simulink model "SG__REF_O_104"  (R2022b)
settings: Solver=FixedStepAuto  StartTime=0.0  StopTime=Inf  RelTol=1e-3  EnableMultiTasking=on
model workspace (MAT data in the model file):
  N_trig = Simulink.Parameter
  N_trig.Value = 4
  N_trig.Description = 'number of samples for triggered pulse for recording'
  N_trig.DataType = 'auto'
  N_trig.Complexity = 'real'
  N_trig.Dimensions = [1 1]
  a_1 = Simulink.Parameter
  a_1.Value = [1 1 1]
  a_1.DataType = 'auto'
  a_1.Complexity = 'real'
  a_1.Dimensions = [1 3]
  b_1 = Simulink.Parameter
  b_1.Value = [0.5 0.5 0.5]
  b_1.DataType = 'auto'
  b_1.Complexity = 'real'
  b_1.Dimensions = [1 3]
  enable_source = Simulink.Parameter
  enable_source.Value = 0
  enable_source.DataType = 'boolean'
  enable_source.Complexity = 'real'
  enable_source.Dimensions = [1 1]
  freq_fin = Simulink.Parameter
  freq_fin.Value = 1200
  freq_fin.DataType = 'auto'
  freq_fin.Complexity = 'real'
  freq_fin.Dimensions = [1 1]
  freq_ini = Simulink.Parameter
  freq_ini.Value = 150
  freq_ini.DataType = 'auto'
  freq_ini.Complexity = 'real'
  freq_ini.Dimensions = [1 1]
  k_1 = Simulink.Parameter
  k_1.Value = [0 0 0]
  k_1.DataType = 'auto'
  k_1.Complexity = 'real'
  k_1.Dimensions = [1 3]
  rec = Simulink.Parameter
  rec.Value = 0
  rec.DataType = 'boolean'
  rec.Complexity = 'real'
  rec.Dimensions = [1 1]
  src_select = Simulink.Parameter
  src_select.Value = 0
  src_select.DataType = 'auto'
  src_select.Complexity = 'real'
  src_select.Dimensions = [1 1]
  sweep_gain = Simulink.Parameter
  sweep_gain.Value = 0.02
  sweep_gain.DataType = 'auto'
  sweep_gain.Complexity = 'real'
  sweep_gain.Dimensions = [1 1]
  tmax = Simulink.Parameter
  tmax.Value = 10
  tmax.DataType = 'auto'
  tmax.Complexity = 'real'
  tmax.Dimensions = [1 1]
  ts_rec = Simulink.Parameter
  ts_rec.Value = 0.0001
  ts_rec.DataType = 'auto'
  ts_rec.Complexity = 'real'
  ts_rec.Dimensions = [1 1]
undefined symbols (not defined in the file): Ended, Single
libraries: speedgoatlib_IO104 x2
settings Model: SimulationMode=external  DataflowThreadingImplementation=Pthreads  Creator=padlewsk  LastModifiedBy=padlewsk
settings SolverCC: ConcurrentTasks=on  AlgebraicLoopSolver=TrustRegion  PositivePriorityOrder=on  AutoInsertRateTranBlk=on
settings DataIOCC: SaveFormat=StructureWithTime
settings OptimizationCC: GainParamInheritBuiltInType=on  RollThreshold=9  EfficientFloat2IntCast=on  SimCompilerOptimization=on
settings DebuggingCC: TasksWithSamePriorityMsg=none  UnconnectedInputMsg=warning  UnconnectedOutputMsg=warning  UnconnectedLineMsg=warning
settings HardwareCC: ProdBitPerLong=64  ProdLongLongMode=on  ProdHWDeviceType=Intel->x86-64 (Linux 64)
settings ModelReferenceCC: EnableRefExpFcnMdlSchedulingChecks=on  ModelReferenceNumInstancesAllowed=Single
settings RTWCC: Description=Simulink Real-Time  SystemTargetFile=slrealtime.tlc  TemplateMakefile=slrealtime_default_tmf  Toolchain=Simulink Real-Time Toolchain  BuildConfiguration=Faster Runs  CodeExecutionProfiling=on  TargetLang=C++

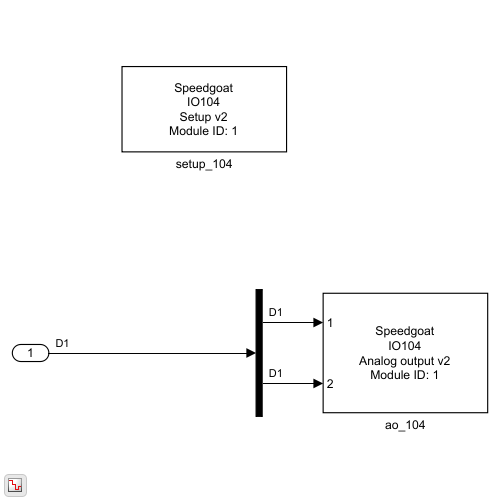
[thumbnail: Simulink's stored preview of the top-level diagram]
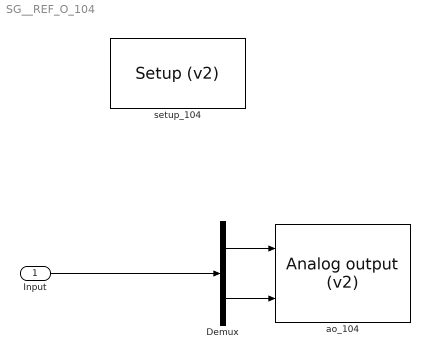
== system SG__REF_O_104 ==
  Input : Inport
  Demux : Demux  Outputs=2
  ao_104 : speedgoatlib_IO104/Analog output (v2)   parModuleId=1  parTs=ts  parPciSlot=-1  parDaSimultaneous=on  parDaChannels=[1,2]  parDaChannelsSorted=[1,2]  parDaInitValue=[0,0]  parDaReset=[1,1]  parDaRange=+-10V  parDaFrameSize=1  parDaUseTrigger=off  parDaClockInitiator=Initiator  parDaSampleTime=9.920634921e-07  parTriggerInitiator=Initiator  parTriggerRate=4.161015625e-01  parAdBlockPresent=0
      settings: SourceProductName=Simulink Real-Time: Speedgoat I/O Blockset
  setup_104 : speedgoatlib_IO104/Setup (v2)   parPciSlot=-1  parModuleId=1  parTriggerInitiator=Initiator  parTriggerRate=4.161015625e-01  parCalibrate=off  parAdChannels=[1:8]  parAdRange1=+-2.5V  parAdRange2=+-2.5V  parAdCoupling=Single-Ended  parAdUseTrigger=off  parAdFrameSize=1  parAdClockInitiator=Initiator  parAdSampleTime=9.920634921e-07  parDaSimultaneous=on  parDaChannels=[1:2]  parDaChannelsSorted=[1,2]  parDaInitValue=[0]  parDaReset=[1]  parDaRange=+-10V  parDaUseTrigger=off  parDaFrameSize=1  parDaClockInitiator=Initiator  parDaSampleTime=9.920634921e-07  parDioByte0Dir=Outputs  parDioByte1Dir=Inputs  parDoChannels=[]  parDoInitValues=[0]  parDoReset=[1]  parDiChannels=[]
      settings: SourceProductName=Simulink Real-Time: Speedgoat I/O Blockset
  wires:
  Demux/1 -> ao_104/1
  Demux/2 -> ao_104/2
  Input/1 -> Demux/1
